simulink model "Cruisecontrol"  (R2020a)
settings: Solver=VariableStepAuto  StartTime=0.0  StopTime=10.0  RelTol=1e-3
values from neighbouring files (symbols this model uses):
  b = 50    [workspace_data.mat]
  m = 1000    [workspace_data.mat]
settings Model: Creator=shweta  LastModifiedBy=shweta

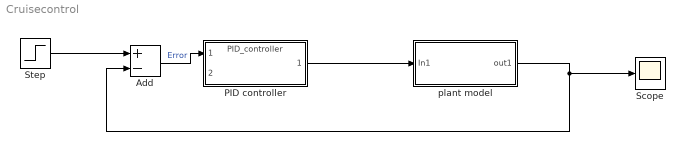
== system Cruisecontrol ==
  Add : Sum  Inputs=+-
  PID controller : ModelReference  ModelNameDialog=PID_controller  SimulationMode=Normal  ModelReferenceVersion=1.1
  Scope : Scope
  Step : Step  Time=0  SampleTime=0
  plant model : Subsystem
  wires:
  PID controller/1 -> plant model/1(In1)
  plant model/1(out1) -> Scope/1, Add/2
  Step/1 -> Add/1
  Add/1 -> PID controller/1  "Error"

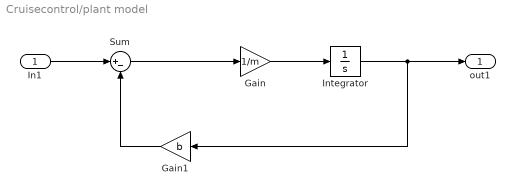
== system Cruisecontrol/plant model ==
  In1 : Inport
  Gain : Gain  Gain=1/m
  Gain1 : Gain  Gain=b
  Integrator : Integrator
  Sum : Sum  Inputs=|+-
  out1 : Outport
  wires:
  Integrator/1 -> Gain1/1, out1/1
  Sum/1 -> Gain/1
  Gain1/1 -> Sum/2
  Gain/1 -> Integrator/1
  In1/1 -> Sum/1
